simulink model "pv_boost_mpp_Iref"  (Simulink 6.5)
settings: Solver=ode45  StartTime=0.0  StopTime=60*8  MaxStep=0.1  RelTol=1e-3
libraries: simulink x11
settings Model: Creator=Mama  LastModifiedBy=Mama
settings SolverCC: MaxConsecutiveMinStep=2
settings DebuggingCC: AlgebraicLoopMsg=none  SolverPrmCheckMsg=none  UnconnectedOutputMsg=none

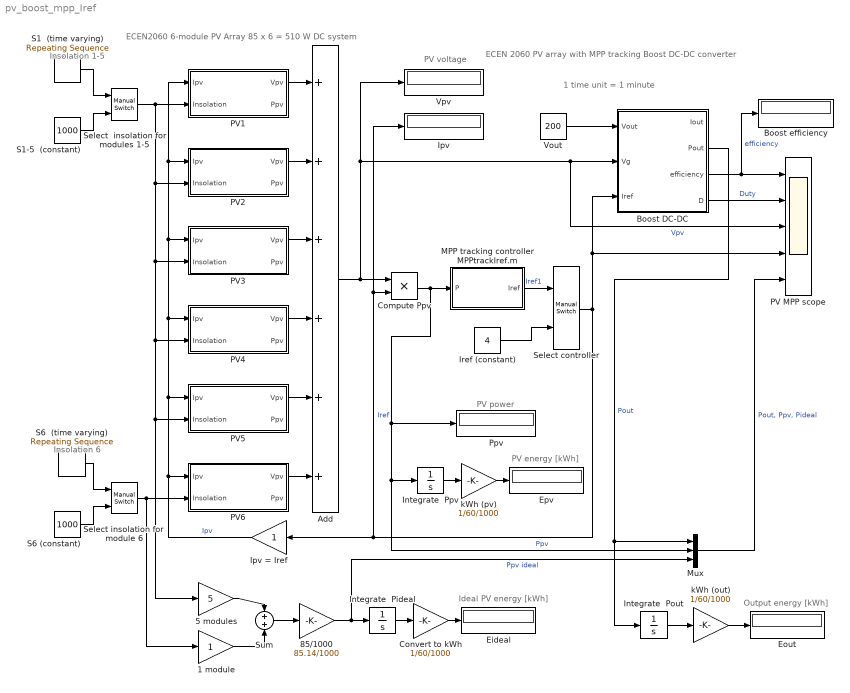
== system pv_boost_mpp_Iref ==
  note: ECEN2060
      | 6-module PV Array
      | 85 x 6 = 510 W DC system
  note: Insolation 1-5
  note: Insolation 6
  note: PV power
  note: PV energy [kWh]
  note: Ideal PV energy [kWh]
  note: ECEN 2060 PV array with
      | MPP tracking
      | Boost DC-DC converter
  note: 1 time unit = 1 minute
  note: PV voltage
  note: Output energy [kWh]
  1 module : Gain
  5 modules : Gain  Gain=5
  85/1000 : Gain  Gain=85.14/1000
  Add : Sum  Inputs=++++++  OutScaling=2^-10
  Boost DC-DC : Subsystem  mask{RL=0.5, Isw=0.03}
      mask prompts: RL "Input port series resistance RL"; Isw "Switching loss current Isw"
      mask help: Averaged model of a boost (step-up) DC-DC converter with input current control. Model includes RL (conduction loss model) in series with the input port and Isw (model of switching and other loss) in parallel with the output port
      mask Display:
      | text(0.5,0.9,'Boost','horizontalAlignment', 'center');
      | text(0.5,0.8,'DC-DC','horizontalAlignment', 'center');
      | text(0.5,0.7,'(averaged)','horizontalAlignment', 'center');
      | text(0.5,0.6,'Iref control','horizontalAlignment', 'center');
  Boost efficiency : Display
  Compute Ppv : Product  RndMeth=Zero
  Convert to kWh : Gain  Gain=1/60/1000
  Eideal : Display
  Eout : Display
  Epv : Display
  Integrate  Pideal : Integrator
  Integrate  Pout : Integrator
  Integrate  Ppv : Integrator
  Ipv : Display
  Ipv = Iref : Gain  Orientation=left
  Iref (constant) : Constant  Value=4  OutDataType=sfix(16)  ConRadixGroup=Use specified scaling  OutScaling=2^0  SampleTime=inf  FramePeriod=inf
  MPP tracking controller MPPtrackIref.m : Subsystem  mask{Tsample=0.2}
      mask prompts: Tsample "Sample interval"
      mask init:
      | InitializeMPPtrackIref
      mask Display: text(0.5,0.5,'MPPT','horizontalAlignment', 'center');
  Mux : Mux  Inputs=3
  PV MPP scope : Scope  NumInputPorts=5
      settings: TimeRange=500  YMin=0~0.4~-50~0~-500  YMax=1~1~150~6~1000
  PV1 : Subsystem  mask{Isc=5.45, Voc=22.2, Ir=4.95, Vr=17.2, Diode=on}
      mask prompts: Isc "Short-circuit current"; Voc "Open-circuit voltage"; Ir "Current at Pmax"; Vr "Voltage at Pmax"; Diode "By-pass diode?"
      mask help: PV module model based on module data-sheet parameters. This model has Ipv input, which is suitable for series connections. Limitations: no temperature dependance, static model
      mask init:
      | % calculation of PV module parameters
      | % limitation: constant temperature
      | Ns = round(Voc/0.61); % default number of cells in series
      | Vt = 26e-3; % thermal voltage
      | G = Isc/1000; % irradiation to short-circuit current gain
      | Vmpc = Vr/Ns; % cell voltage at rated Pmax
      | Vocc = Voc/Ns; % cell open-circuit voltage
      | Rmpp = Vmpc/Ir; % cell load resistance at Pmax
      | %
      | Rp = 100*Vocc/Isc; % initial value for Rp
      | Vdm = Vocc; % initial value for Vdm
      | %
      | % iterative solution for model parameters: Io, Rs, Rp
      | for i=1:10
      | %
      |  Idm = Isc - Ir - Vdm/Rp; % pn-junction (diode) current at MPP
      |  Io = (Isc-Vocc/Rp)/(exp(Vocc/Vt)-1); % pn-junction reverse saturation current
      |  Vdm = Vt*log(Idm/Io+1); % pn-junction (diode) voltage at MPP
      |  Rs = (Vdm-Vmpc)/Ir; % cell series resistance
      |  Rd = (Rmpp - Rs)*Rp/(Rp-Rmpp+Rs); % diode incremental resistance at MPP
      |  Idm = Vt/Rd; % diode current at MPP based on incremental resistance
      |  Rp = Vdm/(Isc-Ir-Idm); % cell parallel resistance
      | %
      | end
      | %
      mask Display:
      | plot([0.3 0.4],[0.4 0.8]);
      | plot([0.4 0.5],[0.4 0.8]);
      | plot([0.5 0.6],[0.4 0.8]);
      | plot([0.6 0.7],[0.4 0.8]);
      | plot([0.3 0.6],[0.4 0.4]);
      | plot([0.325 0.625],[0.5 0.5]);
      | plot([0.35 0.65],[0.6 0.6]);
      | plot([0.375 0.675],[0.7 0.7]);
      | plot([0.4 0.7],[0.8 0.8]);
      | text(0.5,0.9,'PV module (I)','horizontalAlignment', 'center');
  PV2 : Subsystem  mask{Isc=5.45, Voc=22.2, Ir=4.95, Vr=17.2, Diode=on}
      mask prompts: Isc "Short-circuit current"; Voc "Open-circuit voltage"; Ir "Current at Pmax"; Vr "Voltage at Pmax"; Diode "By-pass diode?"
      mask help: PV module model based on module data-sheet parameters. This model has Ipv input, which is suitable for series connections. Limitations: no temperature dependance, static model
      mask init: same as pv_boost_mpp_Iref/PV1
      mask Display:
      | plot([0.3 0.4],[0.4 0.8]);
      | plot([0.4 0.5],[0.4 0.8]);
      | plot([0.5 0.6],[0.4 0.8]);
      | plot([0.6 0.7],[0.4 0.8]);
      | plot([0.3 0.6],[0.4 0.4]);
      | plot([0.325 0.625],[0.5 0.5]);
      | plot([0.35 0.65],[0.6 0.6]);
      | plot([0.375 0.675],[0.7 0.7]);
      | plot([0.4 0.7],[0.8 0.8]);
      | text(0.5,0.9,'PV module (I)','horizontalAlignment', 'center');
  PV3 : Subsystem  mask{Isc=5.45, Voc=22.2, Ir=4.95, Vr=17.2, Diode=on}
      mask prompts: Isc "Short-circuit current"; Voc "Open-circuit voltage"; Ir "Current at Pmax"; Vr "Voltage at Pmax"; Diode "By-pass diode?"
      mask help: PV module model based on module data-sheet parameters. This model has Ipv input, which is suitable for series connections. Limitations: no temperature dependance, static model
      mask init: same as pv_boost_mpp_Iref/PV1
      mask Display:
      | plot([0.3 0.4],[0.4 0.8]);
      | plot([0.4 0.5],[0.4 0.8]);
      | plot([0.5 0.6],[0.4 0.8]);
      | plot([0.6 0.7],[0.4 0.8]);
      | plot([0.3 0.6],[0.4 0.4]);
      | plot([0.325 0.625],[0.5 0.5]);
      | plot([0.35 0.65],[0.6 0.6]);
      | plot([0.375 0.675],[0.7 0.7]);
      | plot([0.4 0.7],[0.8 0.8]);
      | text(0.5,0.9,'PV module (I)','horizontalAlignment', 'center');
  PV4 : Subsystem  mask{Isc=5.45, Voc=22.2, Ir=4.95, Vr=17.2, Diode=on}
      mask prompts: Isc "Short-circuit current"; Voc "Open-circuit voltage"; Ir "Current at Pmax"; Vr "Voltage at Pmax"; Diode "By-pass diode?"
      mask help: PV module model based on module data-sheet parameters. This model has Ipv input, which is suitable for series connections. Limitations: no temperature dependance, static model
      mask init: same as pv_boost_mpp_Iref/PV1
      mask Display:
      | plot([0.3 0.4],[0.4 0.8]);
      | plot([0.4 0.5],[0.4 0.8]);
      | plot([0.5 0.6],[0.4 0.8]);
      | plot([0.6 0.7],[0.4 0.8]);
      | plot([0.3 0.6],[0.4 0.4]);
      | plot([0.325 0.625],[0.5 0.5]);
      | plot([0.35 0.65],[0.6 0.6]);
      | plot([0.375 0.675],[0.7 0.7]);
      | plot([0.4 0.7],[0.8 0.8]);
      | text(0.5,0.9,'PV module (I)','horizontalAlignment', 'center');
  PV5 : Subsystem  mask{Isc=5.45, Voc=22.2, Ir=4.95, Vr=17.2, Diode=on}
      mask prompts: Isc "Short-circuit current"; Voc "Open-circuit voltage"; Ir "Current at Pmax"; Vr "Voltage at Pmax"; Diode "By-pass diode?"
      mask help: PV module model based on module data-sheet parameters. This model has Ipv input, which is suitable for series connections. Limitations: no temperature dependance, static model
      mask init: same as pv_boost_mpp_Iref/PV1
      mask Display:
      | plot([0.3 0.4],[0.4 0.8]);
      | plot([0.4 0.5],[0.4 0.8]);
      | plot([0.5 0.6],[0.4 0.8]);
      | plot([0.6 0.7],[0.4 0.8]);
      | plot([0.3 0.6],[0.4 0.4]);
      | plot([0.325 0.625],[0.5 0.5]);
      | plot([0.35 0.65],[0.6 0.6]);
      | plot([0.375 0.675],[0.7 0.7]);
      | plot([0.4 0.7],[0.8 0.8]);
      | text(0.5,0.9,'PV module (I)','horizontalAlignment', 'center');
  PV6 : Subsystem  mask{Isc=5.45, Voc=22.2, Ir=4.95, Vr=17.2, Diode=on}
      mask prompts: Isc "Short-circuit current"; Voc "Open-circuit voltage"; Ir "Current at Pmax"; Vr "Voltage at Pmax"; Diode "By-pass diode?"
      mask help: PV module model based on module data-sheet parameters. This model has Ipv input, which is suitable for series connections. Limitations: no temperature dependance, static model
      mask init: same as pv_boost_mpp_Iref/PV1
      mask Display:
      | plot([0.3 0.4],[0.4 0.8]);
      | plot([0.4 0.5],[0.4 0.8]);
      | plot([0.5 0.6],[0.4 0.8]);
      | plot([0.6 0.7],[0.4 0.8]);
      | plot([0.3 0.6],[0.4 0.4]);
      | plot([0.325 0.625],[0.5 0.5]);
      | plot([0.35 0.65],[0.6 0.6]);
      | plot([0.375 0.675],[0.7 0.7]);
      | plot([0.4 0.7],[0.8 0.8]);
      | text(0.5,0.9,'PV module (I)','horizontalAlignment', 'center');
  Ppv : Display
  S1  (time varying) : simulink/Sources/Repeating Sequence  SystemSampleTime=-1  rep_seq_t=[0 1*60 2*60 3*60 4*60 5*60 6*60 7*60 8*60]  rep_seq_y=[0 400 850 950 1000 950 850 400 0]
  S1-5  (constant) : Constant  Value=1000  OutDataType=sfix(16)  ConRadixGroup=Use specified scaling  OutScaling=2^0  SampleTime=inf  FramePeriod=inf
  S6  (time varying) : simulink/Sources/Repeating Sequence  SystemSampleTime=-1  rep_seq_t=[0 1*60 2*60 3*60 4*60 5*60 6*60 7*60 8*60]  rep_seq_y=[0 400 850 950 0 950 850 400 0]
  S6 (constant) : Constant  Value=1000  OutDataType=sfix(16)  ConRadixGroup=Use specified scaling  OutScaling=2^0  SampleTime=inf  FramePeriod=inf
  Select controller : simulink/Signal Routing/Manual Switch  SystemSampleTime=-1  sw=1  action=0
  Select insolation for  module 6 : simulink/Signal Routing/Manual Switch  SystemSampleTime=-1  sw=0  action=0
  Select  insolation for modules 1-5 : simulink/Signal Routing/Manual Switch  SystemSampleTime=-1  sw=0  action=0
  Sum : Sum  Inputs=+|+
  Vout : Constant  Value=200  OutDataType=sfix(16)  ConRadixGroup=Use specified scaling  OutScaling=2^0  SampleTime=inf  FramePeriod=inf
  Vpv : Display
  kWh (out) : Gain  Gain=1/60/1000
  kWh (pv) : Gain  Gain=1/60/1000
  wires:
  PV1/1(Vpv) -> Add/1
  PV2/1(Vpv) -> Add/2
  PV3/1(Vpv) -> Add/3
  PV4/1(Vpv) -> Add/4
  PV5/1(Vpv) -> Add/5
  PV6/1(Vpv) -> Add/6
  Vout/1 -> Boost DC-DC/1(Vout)
  Ipv = Iref/1 -> PV1/1(Ipv), PV2/1(Ipv), PV3/1(Ipv), PV4/1(Ipv), PV5/1(Ipv), PV6/1(Ipv)  "Ipv"
  Select  insolation for modules 1-5/1 -> PV1/2(Insolation), PV2/2(Insolation), PV3/2(Insolation), PV4/2(Insolation), PV5/2(Insolation), 5 modules/1
  S1  (time varying)/1 -> Select  insolation for modules 1-5/1
  S1-5  (constant)/1 -> Select  insolation for modules 1-5/2
  S6 (constant)/1 -> Select insolation for  module 6/2
  Select insolation for  module 6/1 -> PV6/2(Insolation), 1 module/1
  Add/1 -> Compute Ppv/1, Vpv/1, Boost DC-DC/2(Vg), PV MPP scope/3  "Vpv"
  Compute Ppv/1 -> MPP tracking controller MPPtrackIref.m/1(P), Ppv/1, Integrate  Ppv/1, Mux/2  "Ppv"
  MPP tracking controller MPPtrackIref.m/1(Iref) -> Select controller/1  "Iref1"
  Iref (constant)/1 -> Select controller/2
  Select controller/1 -> Ipv = Iref/1, Compute Ppv/2, Ipv/1, Boost DC-DC/3(Iref), PV MPP scope/4  "Iref"
  kWh (pv)/1 -> Epv/1
  Integrate  Ppv/1 -> kWh (pv)/1
  Boost DC-DC/2(Pout) -> Mux/1, Integrate  Pout/1  "Pout"
  5 modules/1 -> Sum/1
  1 module/1 -> Sum/2
  Sum/1 -> 85/1000/1
  85/1000/1 -> Integrate  Pideal/1, Mux/3  "Ppv ideal"
  Integrate  Pideal/1 -> Convert to kWh/1
  Convert to kWh/1 -> Eideal/1
  Mux/1 -> PV MPP scope/5  "Pout, Ppv, Pideal"
  Boost DC-DC/4(D) -> PV MPP scope/2  "Duty"
  Boost DC-DC/3(efficiency) -> Boost efficiency/1, PV MPP scope/1  "efficiency"
  S6  (time varying)/1 -> Select insolation for  module 6/1
  Integrate  Pout/1 -> kWh (out)/1
  kWh (out)/1 -> Eout/1

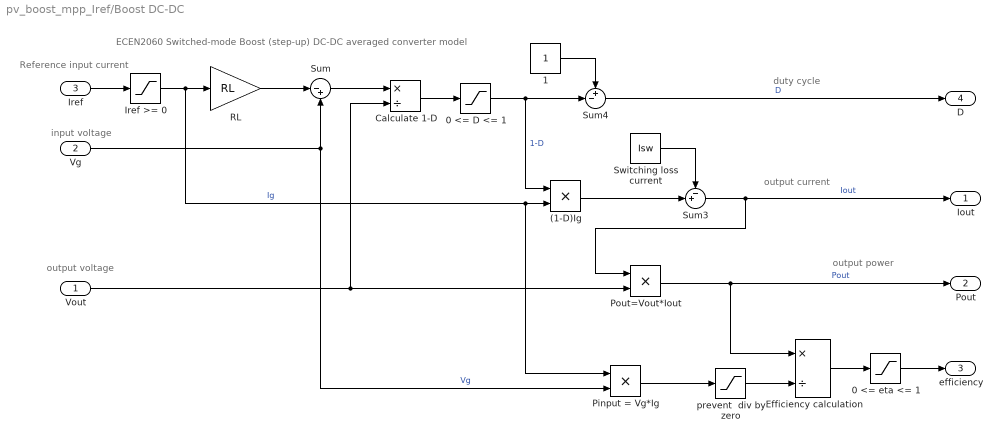
== system pv_boost_mpp_Iref/Boost DC-DC ==
  note: ECEN2060 Switched-mode Boost (step-up) DC-DC averaged converter model
  note: output current
  note: output voltage
  note: input voltage
  note: Reference
      | input current
  note: duty cycle
  note: output power
  Vout : Inport
  Vg : Inport  Port=2
  Iref : Inport  Port=3
  (1-D)Ig : Product  Inputs=**  RndMeth=Zero
  0 <= D <= 1 : Saturate  UpperLimit=1  LowerLimit=0
  0 <= eta <= 1 : Saturate  UpperLimit=1  LowerLimit=0
  1 : Constant  Value=1  OutDataType=sfix(16)  ConRadixGroup=Use specified scaling  OutScaling=2^0  SampleTime=inf  FramePeriod=inf
  Calculate 1-D : Product  Inputs=*/  RndMeth=Zero
  Efficiency calculation : Product  Inputs=*/  RndMeth=Zero
  Iref >= 0 : Saturate  UpperLimit=inf  LowerLimit=0
  Pinput = Vg*Ig : Product  Inputs=**  RndMeth=Zero
  Pout=Vout*Iout : Product  Inputs=**  RndMeth=Zero
  RL : Gain  Gain=RL
  Sum : Sum  Inputs=|-+
  Sum3 : Sum  Inputs=-+|
  Sum4 : Sum  Inputs=+-|
  Switching loss current : Constant  Value=Isw  OutDataType=sfix(16)  ConRadixGroup=Use specified scaling  OutScaling=2^0  SampleTime=inf  FramePeriod=inf
  prevent  div by zero : Saturate  UpperLimit=inf  LowerLimit=eps
  Iout : Outport
  Pout : Outport  Port=2
  efficiency : Outport  Port=3
  D : Outport  Port=4
  wires:
  Efficiency calculation/1 -> 0 <= eta <= 1/1
  Iref/1 -> Iref >= 0/1
  Vout/1 -> Pout=Vout*Iout/2, Calculate 1-D/2
  Switching loss current/1 -> Sum3/1
  Sum3/1 -> Iout/1, Pout=Vout*Iout/1  "Iout"
  Pout=Vout*Iout/1 -> Pout/1, Efficiency calculation/1  "Pout"
  0 <= eta <= 1/1 -> efficiency/1
  Iref >= 0/1 -> RL/1, (1-D)Ig/2, Pinput = Vg*Ig/1  "Ig"
  RL/1 -> Sum/1
  Vg/1 -> Sum/2, Pinput = Vg*Ig/2  "Vg"
  Sum/1 -> Calculate 1-D/1
  Calculate 1-D/1 -> 0 <= D <= 1/1
  0 <= D <= 1/1 -> Sum4/2, (1-D)Ig/1  "1-D"
  1/1 -> Sum4/1
  Sum4/1 -> D/1  "D"
  (1-D)Ig/1 -> Sum3/2
  prevent  div by zero/1 -> Efficiency calculation/2
  Pinput = Vg*Ig/1 -> prevent  div by zero/1

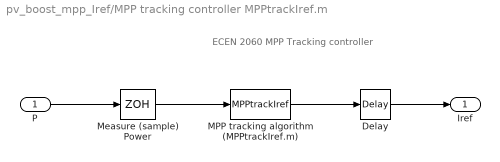
== system pv_boost_mpp_Iref/MPP tracking controller MPPtrackIref.m ==
  note: ECEN 2060 MPP Tracking controller
  P : Inport
  Delay : TransportDelay  DelayTime=Tsample/2
  MPP tracking algorithm (MPPtrackIref.m) : MATLABFcn  MATLABFcn=MPPtrackIref
  Measure (sample) Power : ZeroOrderHold  SampleTime=Tsample
  Iref : Outport
  wires:
  P/1 -> Measure (sample) Power/1
  Measure (sample) Power/1 -> MPP tracking algorithm (MPPtrackIref.m)/1
  MPP tracking algorithm (MPPtrackIref.m)/1 -> Delay/1
  Delay/1 -> Iref/1

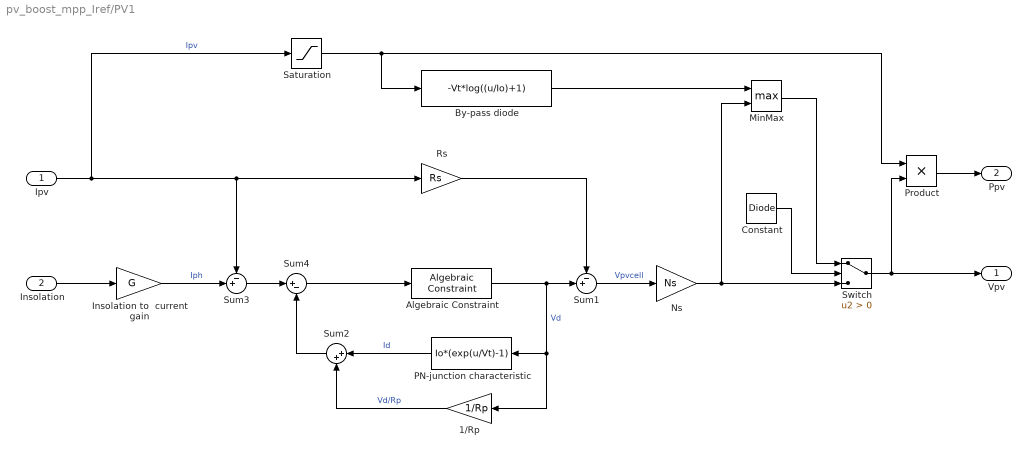
== system pv_boost_mpp_Iref/PV1 ==
  Ipv : Inport
  Insolation : Inport  Port=2
  1/Rp : Gain  Orientation=left  Gain=1/Rp
  Algebraic Constraint : simulink/Math Operations/Algebraic Constraint  SystemSampleTime=-1  z0=0
  By-pass diode : Fcn  Expr=-Vt*log((u/Io)+1)
  Constant : Constant  Value=Diode  OutDataType=sfix(16)  ConRadixGroup=Use specified scaling  OutScaling=2^0  SampleTime=inf  FramePeriod=inf
  Insolation to  current gain : Gain  Gain=G
  MinMax : MinMax  Function=max  Inputs=2
  Ns : Gain  Gain=Ns
  PN-junction characteristic : Fcn  Orientation=left  Expr=Io*(exp(u/Vt)-1)
  Product : Product  RndMeth=Zero
  Rs : Gain  Gain=Rs
  Saturation : Saturate  UpperLimit=inf  LowerLimit=0
  Sum1 : Sum  Inputs=-+|
  Sum2 : Sum  Orientation=left  Inputs=|++
  Sum3 : Sum  Inputs=-+|
  Sum4 : Sum  Inputs=|+-
  Switch : Switch  Criteria=u2 > Threshold
  Vpv : Outport
  Ppv : Outport  Port=2
  wires:
  Insolation/1 -> Insolation to  current gain/1
  Insolation to  current gain/1 -> Sum3/2  "Iph"
  Ipv/1 -> Saturation/1, Sum3/1, Rs/1  "Ipv"
  Product/1 -> Ppv/1
  Sum4/1 -> Algebraic Constraint/1
  Algebraic Constraint/1 -> Sum1/2, 1/Rp/1, PN-junction characteristic/1  "Vd"
  Sum1/1 -> Ns/1  "Vpvcell"
  Rs/1 -> Sum1/1
  By-pass diode/1 -> MinMax/1
  Ns/1 -> MinMax/2, Switch/3
  MinMax/1 -> Switch/1
  Constant/1 -> Switch/2
  Switch/1 -> Vpv/1, Product/2
  Saturation/1 -> Product/1, By-pass diode/1
  Sum3/1 -> Sum4/1
  Sum2/1 -> Sum4/2
  PN-junction characteristic/1 -> Sum2/1  "Id"
  1/Rp/1 -> Sum2/2  "Vd/Rp"

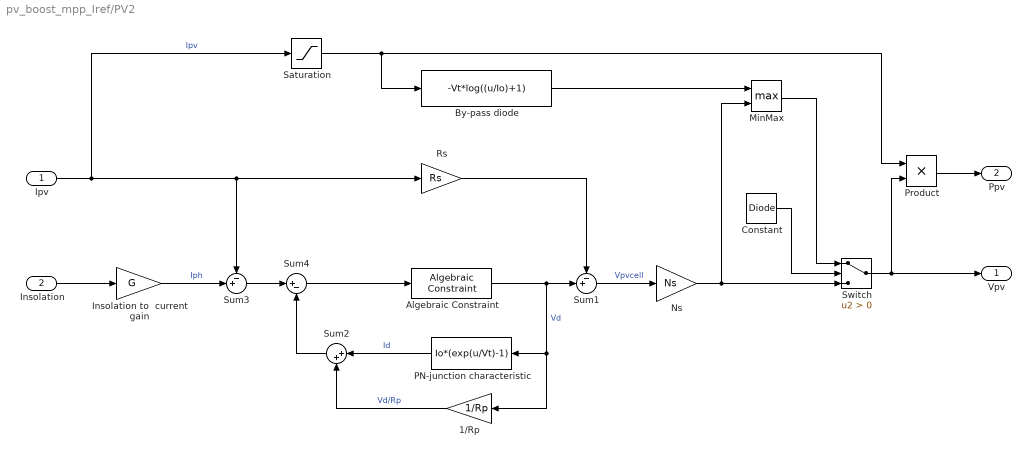
== system pv_boost_mpp_Iref/PV2 ==
  Ipv : Inport
  Insolation : Inport  Port=2
  1/Rp : Gain  Orientation=left  Gain=1/Rp
  Algebraic Constraint : simulink/Math Operations/Algebraic Constraint  SystemSampleTime=-1  z0=0
  By-pass diode : Fcn  Expr=-Vt*log((u/Io)+1)
  Constant : Constant  Value=Diode  OutDataType=sfix(16)  ConRadixGroup=Use specified scaling  OutScaling=2^0  SampleTime=inf  FramePeriod=inf
  Insolation to  current gain : Gain  Gain=G
  MinMax : MinMax  Function=max  Inputs=2
  Ns : Gain  Gain=Ns
  PN-junction characteristic : Fcn  Orientation=left  Expr=Io*(exp(u/Vt)-1)
  Product : Product  RndMeth=Zero
  Rs : Gain  Gain=Rs
  Saturation : Saturate  UpperLimit=inf  LowerLimit=0
  Sum1 : Sum  Inputs=-+|
  Sum2 : Sum  Orientation=left  Inputs=|++
  Sum3 : Sum  Inputs=-+|
  Sum4 : Sum  Inputs=|+-
  Switch : Switch  Criteria=u2 > Threshold
  Vpv : Outport
  Ppv : Outport  Port=2
  wires:
  Insolation/1 -> Insolation to  current gain/1
  Insolation to  current gain/1 -> Sum3/2  "Iph"
  Ipv/1 -> Saturation/1, Sum3/1, Rs/1  "Ipv"
  Product/1 -> Ppv/1
  Sum4/1 -> Algebraic Constraint/1
  Algebraic Constraint/1 -> Sum1/2, 1/Rp/1, PN-junction characteristic/1  "Vd"
  Sum1/1 -> Ns/1  "Vpvcell"
  Rs/1 -> Sum1/1
  By-pass diode/1 -> MinMax/1
  Ns/1 -> MinMax/2, Switch/3
  MinMax/1 -> Switch/1
  Constant/1 -> Switch/2
  Switch/1 -> Vpv/1, Product/2
  Saturation/1 -> Product/1, By-pass diode/1
  Sum3/1 -> Sum4/1
  Sum2/1 -> Sum4/2
  PN-junction characteristic/1 -> Sum2/1  "Id"
  1/Rp/1 -> Sum2/2  "Vd/Rp"

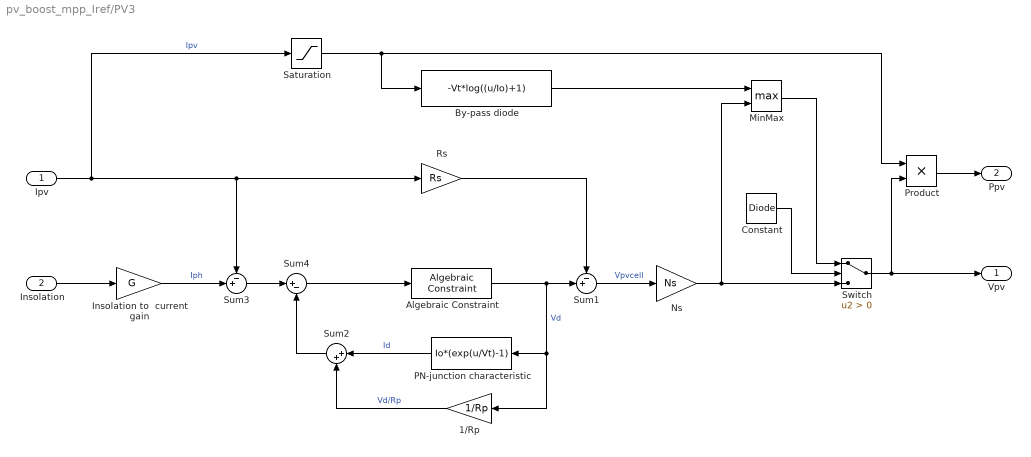
== system pv_boost_mpp_Iref/PV3 ==
  Ipv : Inport
  Insolation : Inport  Port=2
  1/Rp : Gain  Orientation=left  Gain=1/Rp
  Algebraic Constraint : simulink/Math Operations/Algebraic Constraint  SystemSampleTime=-1  z0=0
  By-pass diode : Fcn  Expr=-Vt*log((u/Io)+1)
  Constant : Constant  Value=Diode  OutDataType=sfix(16)  ConRadixGroup=Use specified scaling  OutScaling=2^0  SampleTime=inf  FramePeriod=inf
  Insolation to  current gain : Gain  Gain=G
  MinMax : MinMax  Function=max  Inputs=2
  Ns : Gain  Gain=Ns
  PN-junction characteristic : Fcn  Orientation=left  Expr=Io*(exp(u/Vt)-1)
  Product : Product  RndMeth=Zero
  Rs : Gain  Gain=Rs
  Saturation : Saturate  UpperLimit=inf  LowerLimit=0
  Sum1 : Sum  Inputs=-+|
  Sum2 : Sum  Orientation=left  Inputs=|++
  Sum3 : Sum  Inputs=-+|
  Sum4 : Sum  Inputs=|+-
  Switch : Switch  Criteria=u2 > Threshold
  Vpv : Outport
  Ppv : Outport  Port=2
  wires:
  Insolation/1 -> Insolation to  current gain/1
  Insolation to  current gain/1 -> Sum3/2  "Iph"
  Ipv/1 -> Saturation/1, Sum3/1, Rs/1  "Ipv"
  Product/1 -> Ppv/1
  Sum4/1 -> Algebraic Constraint/1
  Algebraic Constraint/1 -> Sum1/2, 1/Rp/1, PN-junction characteristic/1  "Vd"
  Sum1/1 -> Ns/1  "Vpvcell"
  Rs/1 -> Sum1/1
  By-pass diode/1 -> MinMax/1
  Ns/1 -> MinMax/2, Switch/3
  MinMax/1 -> Switch/1
  Constant/1 -> Switch/2
  Switch/1 -> Vpv/1, Product/2
  Saturation/1 -> Product/1, By-pass diode/1
  Sum3/1 -> Sum4/1
  Sum2/1 -> Sum4/2
  PN-junction characteristic/1 -> Sum2/1  "Id"
  1/Rp/1 -> Sum2/2  "Vd/Rp"

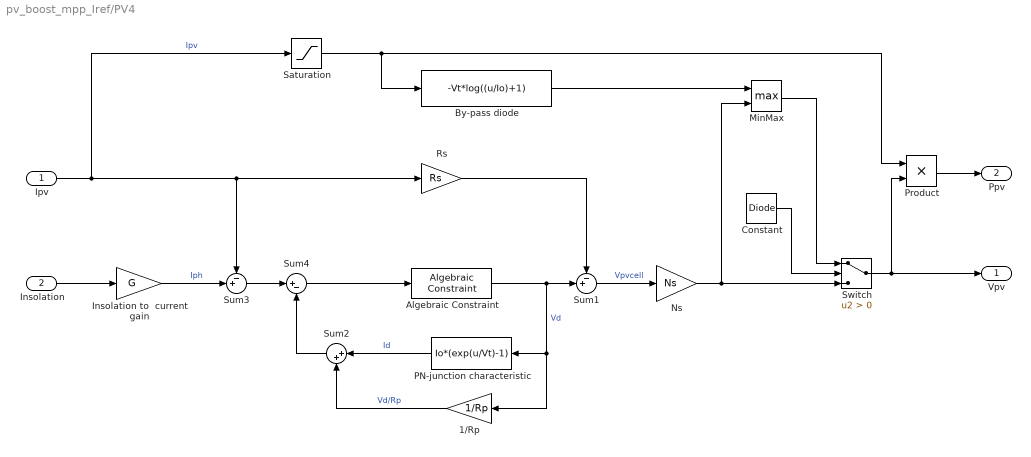
== system pv_boost_mpp_Iref/PV4 ==
  Ipv : Inport
  Insolation : Inport  Port=2
  1/Rp : Gain  Orientation=left  Gain=1/Rp
  Algebraic Constraint : simulink/Math Operations/Algebraic Constraint  SystemSampleTime=-1  z0=0
  By-pass diode : Fcn  Expr=-Vt*log((u/Io)+1)
  Constant : Constant  Value=Diode  OutDataType=sfix(16)  ConRadixGroup=Use specified scaling  OutScaling=2^0  SampleTime=inf  FramePeriod=inf
  Insolation to  current gain : Gain  Gain=G
  MinMax : MinMax  Function=max  Inputs=2
  Ns : Gain  Gain=Ns
  PN-junction characteristic : Fcn  Orientation=left  Expr=Io*(exp(u/Vt)-1)
  Product : Product  RndMeth=Zero
  Rs : Gain  Gain=Rs
  Saturation : Saturate  UpperLimit=inf  LowerLimit=0
  Sum1 : Sum  Inputs=-+|
  Sum2 : Sum  Orientation=left  Inputs=|++
  Sum3 : Sum  Inputs=-+|
  Sum4 : Sum  Inputs=|+-
  Switch : Switch  Criteria=u2 > Threshold
  Vpv : Outport
  Ppv : Outport  Port=2
  wires:
  Insolation/1 -> Insolation to  current gain/1
  Insolation to  current gain/1 -> Sum3/2  "Iph"
  Ipv/1 -> Saturation/1, Sum3/1, Rs/1  "Ipv"
  Product/1 -> Ppv/1
  Sum4/1 -> Algebraic Constraint/1
  Algebraic Constraint/1 -> Sum1/2, 1/Rp/1, PN-junction characteristic/1  "Vd"
  Sum1/1 -> Ns/1  "Vpvcell"
  Rs/1 -> Sum1/1
  By-pass diode/1 -> MinMax/1
  Ns/1 -> MinMax/2, Switch/3
  MinMax/1 -> Switch/1
  Constant/1 -> Switch/2
  Switch/1 -> Vpv/1, Product/2
  Saturation/1 -> Product/1, By-pass diode/1
  Sum3/1 -> Sum4/1
  Sum2/1 -> Sum4/2
  PN-junction characteristic/1 -> Sum2/1  "Id"
  1/Rp/1 -> Sum2/2  "Vd/Rp"

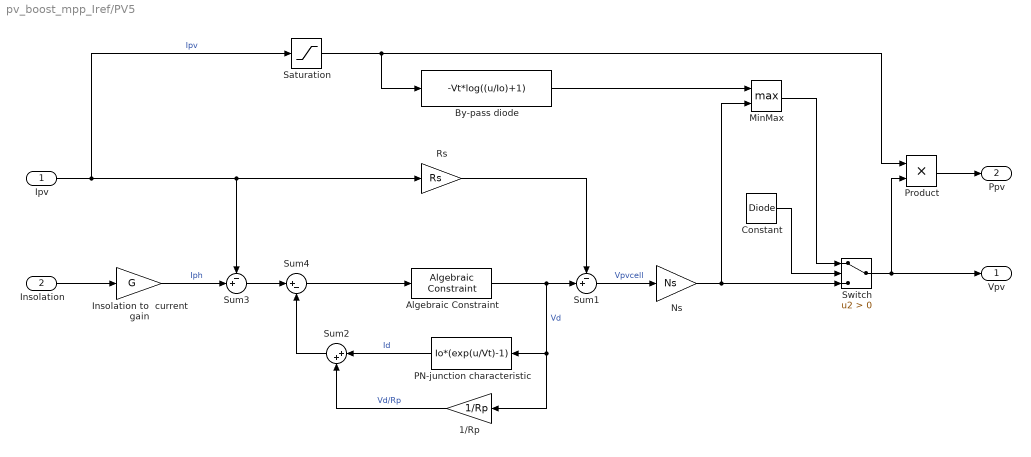
== system pv_boost_mpp_Iref/PV5 ==
  Ipv : Inport
  Insolation : Inport  Port=2
  1/Rp : Gain  Orientation=left  Gain=1/Rp
  Algebraic Constraint : simulink/Math Operations/Algebraic Constraint  SystemSampleTime=-1  z0=0
  By-pass diode : Fcn  Expr=-Vt*log((u/Io)+1)
  Constant : Constant  Value=Diode  OutDataType=sfix(16)  ConRadixGroup=Use specified scaling  OutScaling=2^0  SampleTime=inf  FramePeriod=inf
  Insolation to  current gain : Gain  Gain=G
  MinMax : MinMax  Function=max  Inputs=2
  Ns : Gain  Gain=Ns
  PN-junction characteristic : Fcn  Orientation=left  Expr=Io*(exp(u/Vt)-1)
  Product : Product  RndMeth=Zero
  Rs : Gain  Gain=Rs
  Saturation : Saturate  UpperLimit=inf  LowerLimit=0
  Sum1 : Sum  Inputs=-+|
  Sum2 : Sum  Orientation=left  Inputs=|++
  Sum3 : Sum  Inputs=-+|
  Sum4 : Sum  Inputs=|+-
  Switch : Switch  Criteria=u2 > Threshold
  Vpv : Outport
  Ppv : Outport  Port=2
  wires:
  Insolation/1 -> Insolation to  current gain/1
  Insolation to  current gain/1 -> Sum3/2  "Iph"
  Ipv/1 -> Saturation/1, Sum3/1, Rs/1  "Ipv"
  Product/1 -> Ppv/1
  Sum4/1 -> Algebraic Constraint/1
  Algebraic Constraint/1 -> Sum1/2, 1/Rp/1, PN-junction characteristic/1  "Vd"
  Sum1/1 -> Ns/1  "Vpvcell"
  Rs/1 -> Sum1/1
  By-pass diode/1 -> MinMax/1
  Ns/1 -> MinMax/2, Switch/3
  MinMax/1 -> Switch/1
  Constant/1 -> Switch/2
  Switch/1 -> Vpv/1, Product/2
  Saturation/1 -> Product/1, By-pass diode/1
  Sum3/1 -> Sum4/1
  Sum2/1 -> Sum4/2
  PN-junction characteristic/1 -> Sum2/1  "Id"
  1/Rp/1 -> Sum2/2  "Vd/Rp"

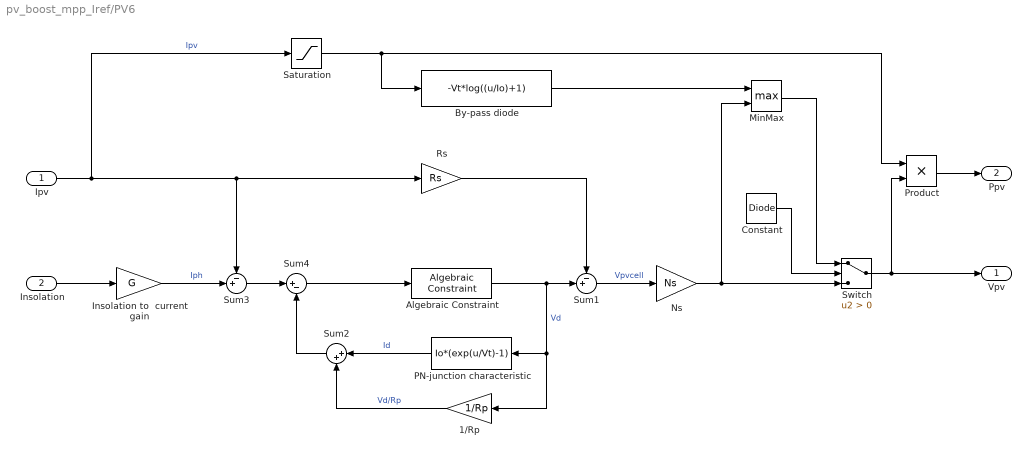
== system pv_boost_mpp_Iref/PV6 ==
  Ipv : Inport
  Insolation : Inport  Port=2
  1/Rp : Gain  Orientation=left  Gain=1/Rp
  Algebraic Constraint : simulink/Math Operations/Algebraic Constraint  SystemSampleTime=-1  z0=0
  By-pass diode : Fcn  Expr=-Vt*log((u/Io)+1)
  Constant : Constant  Value=Diode  OutDataType=sfix(16)  ConRadixGroup=Use specified scaling  OutScaling=2^0  SampleTime=inf  FramePeriod=inf
  Insolation to  current gain : Gain  Gain=G
  MinMax : MinMax  Function=max  Inputs=2
  Ns : Gain  Gain=Ns
  PN-junction characteristic : Fcn  Orientation=left  Expr=Io*(exp(u/Vt)-1)
  Product : Product  RndMeth=Zero
  Rs : Gain  Gain=Rs
  Saturation : Saturate  UpperLimit=inf  LowerLimit=0
  Sum1 : Sum  Inputs=-+|
  Sum2 : Sum  Orientation=left  Inputs=|++
  Sum3 : Sum  Inputs=-+|
  Sum4 : Sum  Inputs=|+-
  Switch : Switch  Criteria=u2 > Threshold
  Vpv : Outport
  Ppv : Outport  Port=2
  wires:
  Insolation/1 -> Insolation to  current gain/1
  Insolation to  current gain/1 -> Sum3/2  "Iph"
  Ipv/1 -> Saturation/1, Sum3/1, Rs/1  "Ipv"
  Product/1 -> Ppv/1
  Sum4/1 -> Algebraic Constraint/1
  Algebraic Constraint/1 -> Sum1/2, 1/Rp/1, PN-junction characteristic/1  "Vd"
  Sum1/1 -> Ns/1  "Vpvcell"
  Rs/1 -> Sum1/1
  By-pass diode/1 -> MinMax/1
  Ns/1 -> MinMax/2, Switch/3
  MinMax/1 -> Switch/1
  Constant/1 -> Switch/2
  Switch/1 -> Vpv/1, Product/2
  Saturation/1 -> Product/1, By-pass diode/1
  Sum3/1 -> Sum4/1
  Sum2/1 -> Sum4/2
  PN-junction characteristic/1 -> Sum2/1  "Id"
  1/Rp/1 -> Sum2/2  "Vd/Rp"
